simulink model "Q4_Simulink"  (R2019b)
settings: Solver=VariableStepAuto  StartTime=0.0  StopTime=simTime  RelTol=1e-3
values from neighbouring files (symbols this model uses):
  atan_scale = 100    [Q6.mat]    (also in Q8.mat)
  b_1 = 0.0029    [Q6.mat]    (also in Q8.mat)
  b_2 = 0.0002    [Q6.mat]    (also in Q8.mat)
  b_3 = 0.00015    [Q6.mat]    (also in Q8.mat)
  C = [1 0 0 0 0 0 0 1 0 0 0 0 ... (18 elements, 3x6)]    [Q6.mat]    (also in Q8.mat)
  f_m = 0.00325471482319    [Q6.mat]
  f_m_time = 5    [Q6.mat]
  J_1 = 0.0025    [Q6.mat]    (also in Q8.mat)
  J_2 = 0.0018    [Q6.mat]    (also in Q8.mat)
  J_3 = 0.0018    [Q6.mat]    (also in Q8.mat)
  k_1 = 2.7    [Q6.mat]    (also in Q8.mat)
  k_2 = 2.6    [Q6.mat]    (also in Q8.mat)
  switch_fault = 1    [Q6.mat]
  T_Cm = 0.0969711017207    [Q6.mat]    (also in Q8.mat)
  T_Cp = 0.0714454263135    [Q6.mat]    (also in Q8.mat)
  T_s = 0.004    [Q6.mat]
  w_th = 0.75    [Q6.mat]    (also in Q8.mat)
  wn = 1    [Q6.mat]
  x_0 = [0 0 0 0 0 0]    [Q6.mat]
  zeta = 0.96    [Q6.mat]
undefined symbols (not defined in the file or in its folder): den_tf_11, den_tf_21, num_tf_11, num_tf_21, sigma_meas
settings Model: Creator=mfust  LastModifiedBy=mfust
settings DataIOCC: ReturnWorkspaceOutputs=off
settings DebuggingCC: ArithmeticOperatorsInVariantConditions=warning
settings SFSimCC: SimUseLocalCustomCode=off  CustomCodeUndefinedFunction=UseInterfaceOnly
settings RTWCC: RTWUseLocalCustomCode=off

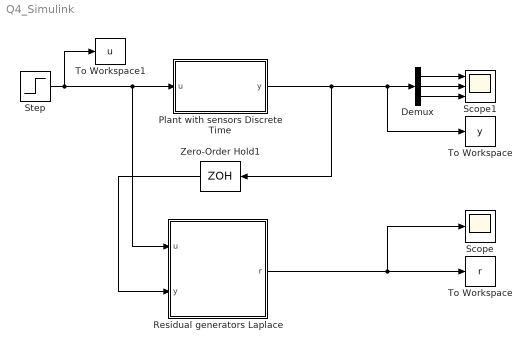
== system Q4_Simulink ==
  Demux : Demux  Outputs=3
  Plant with sensors Discrete Time : Subsystem
  Residual generators Laplace : Subsystem
  Scope : Scope
  Scope1 : Scope  NumInputPorts=3
  Step : Step  Time=2  SampleTime=0
  To Workspace : ToWorkspace  VariableName=y  SaveFormat=Structure With Time  SampleTime=-1
  "To Workspace " : ToWorkspace  VariableName=r  SaveFormat=Structure With Time  SampleTime=-1
  To Workspace1 : ToWorkspace  VariableName=u  SaveFormat=Structure With Time  SampleTime=-1
  Zero-Order Hold1 : ZeroOrderHold  SampleTime=T_s
  wires:
  Residual generators Laplace/1(r) -> Scope/1, "To Workspace "/1
  Step/1 -> Residual generators Laplace/1(u), Plant with sensors Discrete Time/1(u), To Workspace1/1
  Demux/1 -> Scope1/1
  Demux/2 -> Scope1/2
  Demux/3 -> Scope1/3
  Plant with sensors Discrete Time/1(y) -> Zero-Order Hold1/1, To Workspace/1, Demux/1
  Zero-Order Hold1/1 -> Residual generators Laplace/2(y)

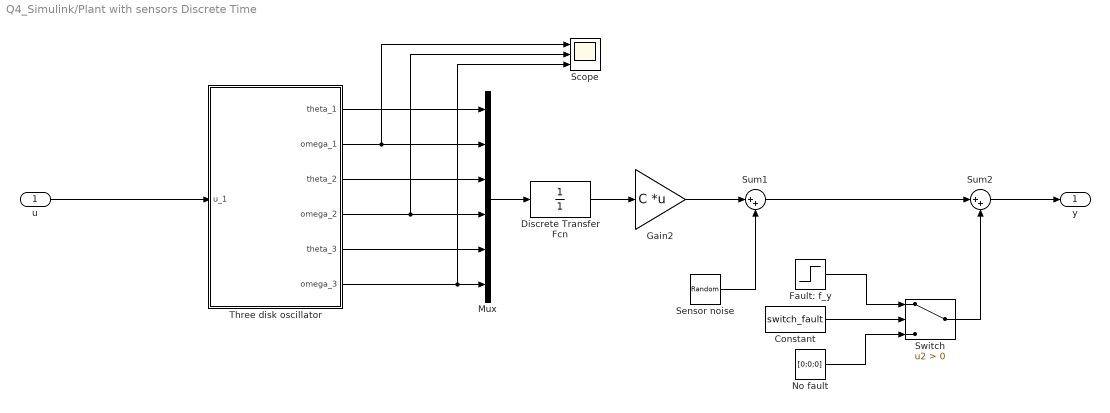
== system Q4_Simulink/Plant with sensors Discrete Time ==
  u : Inport
  Constant : Constant  Value=switch_fault
  Discrete Transfer Fcn : DiscreteTransferFcn  Denominator=[1]  SampleTime=T_s
  Fault: f_y : Step  Time=f_m_time  Before=[0;0;0]  After=f_m  SampleTime=0
  Gain2 : Gain  Gain=C  Multiplication=Matrix(K*u) (u vector)
  Mux : Mux  Inputs=6
  No fault : Constant  Value=[0;0;0]
  Scope : Scope  NumInputPorts=3
  Sensor noise : RandomNumber  Mean=zeros(3,1)  Variance=sigma_meas  SampleTime=T_s
  Sum1 : Sum  Inputs=|++
  Sum2 : Sum  Inputs=|++
  Switch : Switch  Criteria=u2 > Threshold
  Three disk oscillator : Subsystem
  y : Outport  VectorParamsAs1DForOutWhenUnconnected=off
  wires:
  u/1 -> Three disk oscillator/1(u_1)
  Three disk oscillator/2(omega_1) -> Scope/1, Mux/2
  Three disk oscillator/1(theta_1) -> Mux/1
  Mux/1 -> Discrete Transfer Fcn/1
  Three disk oscillator/4(omega_2) -> Scope/2, Mux/4
  Three disk oscillator/3(theta_2) -> Mux/3
  Discrete Transfer Fcn/1 -> Gain2/1
  Sum2/1 -> y/1
  Three disk oscillator/6(omega_3) -> Scope/3, Mux/6
  Three disk oscillator/5(theta_3) -> Mux/5
  Sum1/1 -> Sum2/1
  Gain2/1 -> Sum1/1
  Sensor noise/1 -> Sum1/2
  Switch/1 -> Sum2/2
  Constant/1 -> Switch/2
  Fault: f_y/1 -> Switch/1
  No fault/1 -> Switch/3

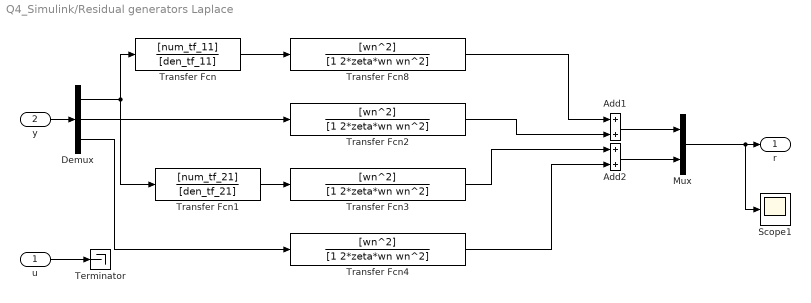
== system Q4_Simulink/Residual generators Laplace ==
  u : Inport
  y : Inport  Port=2
  Add1 : Sum
  Add2 : Sum
  Demux : Demux  Outputs=3
  Mux : Mux  Inputs=2
  Scope1 : Scope
  Terminator : Terminator
  Transfer Fcn : TransferFcn  Numerator=[num_tf_11]  Denominator=[den_tf_11]
  Transfer Fcn1 : TransferFcn  Numerator=[num_tf_21]  Denominator=[den_tf_21]
  Transfer Fcn{2..4,8} (4 alike) : TransferFcn  Numerator=[wn^2]  Denominator=[1 2*zeta*wn wn^2]
  r : Outport  VectorParamsAs1DForOutWhenUnconnected=off
  wires:
  Mux/1 -> Scope1/1, r/1
  y/1 -> Demux/1
  Demux/1 -> Transfer Fcn/1, Transfer Fcn1/1
  u/1 -> Terminator/1
  Add1/1 -> Mux/1
  Add2/1 -> Mux/2
  Transfer Fcn/1 -> Transfer Fcn8/1
  Transfer Fcn8/1 -> Add1/1
  Demux/2 -> Transfer Fcn2/1
  Transfer Fcn2/1 -> Add1/2
  Transfer Fcn1/1 -> Transfer Fcn3/1
  Transfer Fcn3/1 -> Add2/1
  Demux/3 -> Transfer Fcn4/1
  Transfer Fcn4/1 -> Add2/2

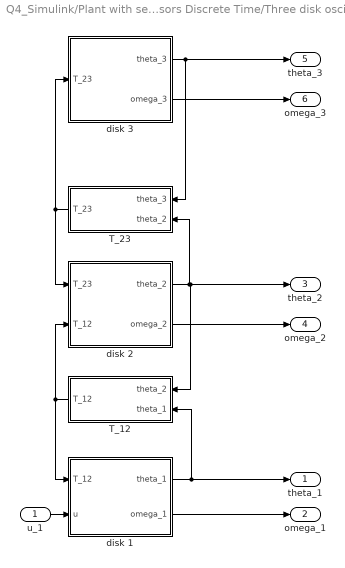
== system Q4_Simulink/Plant with sensors Discrete Time/Three disk oscillator ==
  u_1 : Inport
  T_12 : Subsystem
  T_23 : Subsystem
  disk 1 : Subsystem
  disk 2 : Subsystem
  disk 3 : Subsystem
  theta_1 : Outport  VectorParamsAs1DForOutWhenUnconnected=off
  omega_1 : Outport  Port=2  VectorParamsAs1DForOutWhenUnconnected=off
  theta_2 : Outport  Port=3  VectorParamsAs1DForOutWhenUnconnected=off
  omega_2 : Outport  Port=4  VectorParamsAs1DForOutWhenUnconnected=off
  theta_3 : Outport  Port=5  VectorParamsAs1DForOutWhenUnconnected=off
  omega_3 : Outport  Port=6  VectorParamsAs1DForOutWhenUnconnected=off
  wires:
  T_23/1(T_23) -> disk 2/1(T_23), disk 3/1(T_23)
  disk 1/1(theta_1) -> T_12/2(theta_1), theta_1/1
  disk 2/1(theta_2) -> T_23/2(theta_2), theta_2/1, T_12/1(theta_2)
  T_12/1(T_12) -> disk 1/1(T_12), disk 2/2(T_12)
  disk 3/2(omega_3) -> omega_3/1
  disk 1/2(omega_1) -> omega_1/1
  disk 2/2(omega_2) -> omega_2/1
  u_1/1 -> disk 1/2(u)
  disk 3/1(theta_3) -> theta_3/1, T_23/1(theta_3)

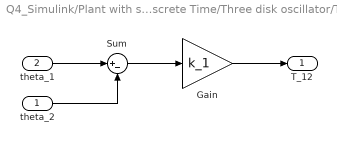
== system Q4_Simulink/Plant with sensors Discrete Time/Three disk oscillator/T_12 ==
  theta_2 : Inport
  theta_1 : Inport  Port=2
  Gain : Gain  Gain=k_1
  Sum : Sum  Inputs=|+-
  T_12 : Outport  VectorParamsAs1DForOutWhenUnconnected=off
  wires:
  theta_2/1 -> Sum/2
  theta_1/1 -> Sum/1
  Sum/1 -> Gain/1
  Gain/1 -> T_12/1

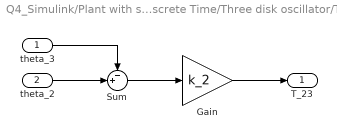
== system Q4_Simulink/Plant with sensors Discrete Time/Three disk oscillator/T_23 ==
  theta_3 : Inport
  theta_2 : Inport  Port=2
  Gain : Gain  Gain=k_2
  Sum : Sum  Inputs=-+|
  T_23 : Outport  VectorParamsAs1DForOutWhenUnconnected=off
  wires:
  Gain/1 -> T_23/1
  Sum/1 -> Gain/1
  theta_3/1 -> Sum/1
  theta_2/1 -> Sum/2

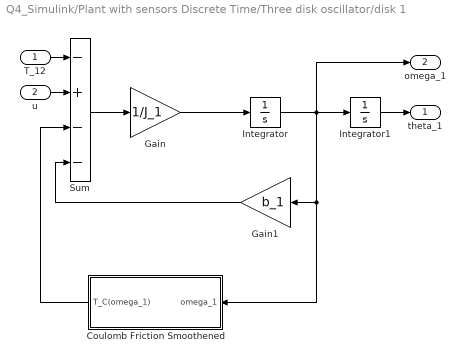
== system Q4_Simulink/Plant with sensors Discrete Time/Three disk oscillator/disk 1 ==
  T_12 : Inport
  u : Inport  Port=2
  Coulomb Friction Smoothened : Subsystem
  Gain : Gain  Gain=1/J_1
  Gain1 : Gain  Gain=b_1
  Integrator : Integrator  InitialCondition=x_0(2)
  Integrator1 : Integrator  InitialCondition=x_0(1)
  Sum : Sum  Inputs=-+--
  theta_1 : Outport  VectorParamsAs1DForOutWhenUnconnected=off
  omega_1 : Outport  Port=2  VectorParamsAs1DForOutWhenUnconnected=off
  wires:
  Sum/1 -> Gain/1
  Integrator/1 -> Integrator1/1, omega_1/1, Coulomb Friction Smoothened/1(omega_1), Gain1/1
  Gain1/1 -> Sum/4
  Integrator1/1 -> theta_1/1
  T_12/1 -> Sum/1
  u/1 -> Sum/2
  Gain/1 -> Integrator/1
  Coulomb Friction Smoothened/1(T_C(omega_1)) -> Sum/3

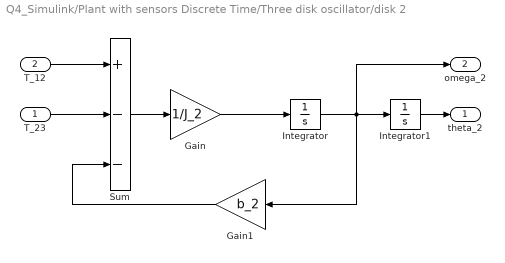
== system Q4_Simulink/Plant with sensors Discrete Time/Three disk oscillator/disk 2 ==
  T_23 : Inport
  T_12 : Inport  Port=2
  Gain : Gain  Gain=1/J_2
  Gain1 : Gain  Gain=b_2
  Integrator : Integrator  InitialCondition=x_0(4)
  Integrator1 : Integrator  InitialCondition=x_0(3)
  Sum : Sum  Inputs=+--
  theta_2 : Outport  VectorParamsAs1DForOutWhenUnconnected=off
  omega_2 : Outport  Port=2  VectorParamsAs1DForOutWhenUnconnected=off
  wires:
  T_23/1 -> Sum/2
  T_12/1 -> Sum/1
  Integrator1/1 -> theta_2/1
  Gain1/1 -> Sum/3
  Gain/1 -> Integrator/1
  Integrator/1 -> Integrator1/1, Gain1/1, omega_2/1
  Sum/1 -> Gain/1

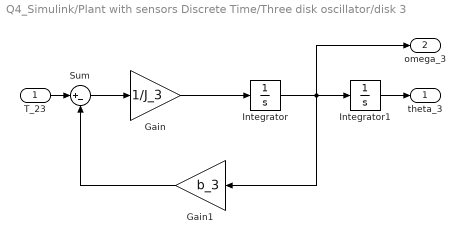
== system Q4_Simulink/Plant with sensors Discrete Time/Three disk oscillator/disk 3 ==
  T_23 : Inport
  Gain : Gain  Gain=1/J_3
  Gain1 : Gain  Gain=b_3
  Integrator : Integrator  InitialCondition=x_0(6)
  Integrator1 : Integrator  InitialCondition=x_0(5)
  Sum : Sum  Inputs=|+-
  theta_3 : Outport  VectorParamsAs1DForOutWhenUnconnected=off
  omega_3 : Outport  Port=2  VectorParamsAs1DForOutWhenUnconnected=off
  wires:
  Sum/1 -> Gain/1
  Integrator/1 -> Integrator1/1, omega_3/1, Gain1/1
  Gain/1 -> Integrator/1
  Gain1/1 -> Sum/2
  Integrator1/1 -> theta_3/1
  T_23/1 -> Sum/1

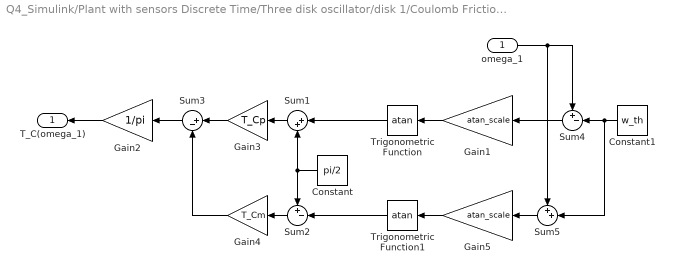
== system Q4_Simulink/Plant with sensors Discrete Time/Three disk oscillator/disk 1/Coulomb Friction Smoothened ==
  omega_1 : Inport
  Constant : Constant  Value=pi/2
  Constant1 : Constant  Value=w_th
  Gain1 : Gain  Gain=atan_scale
  Gain2 : Gain  Gain=1/pi
  Gain3 : Gain  Gain=T_Cp
  Gain4 : Gain  Gain=T_Cm
  Gain5 : Gain  Gain=atan_scale
  Sum1 : Sum  Inputs=|++
  Sum2 : Sum  Inputs=+-|
  Sum3 : Sum  Inputs=|+-
  Sum4 : Sum  Inputs=+-|
  Sum5 : Sum  Inputs=++|
  Trigonometric Function : Trigonometry  Operator=atan
  Trigonometric Function1 : Trigonometry  Operator=atan
  T_C(omega_1) : Outport  VectorParamsAs1DForOutWhenUnconnected=off
  wires:
  Gain1/1 -> Trigonometric Function/1
  Sum1/1 -> Gain3/1
  Constant/1 -> Sum2/1, Sum1/2
  Sum2/1 -> Gain4/1
  Sum3/1 -> Gain2/1
  Trigonometric Function/1 -> Sum1/1
  Gain4/1 -> Sum3/2
  Gain2/1 -> T_C(omega_1)/1
  omega_1/1 -> Sum5/1, Sum4/1
  Gain3/1 -> Sum3/1
  Sum4/1 -> Gain1/1
  Constant1/1 -> Sum5/2, Sum4/2
  Gain5/1 -> Trigonometric Function1/1
  Sum5/1 -> Gain5/1
  Trigonometric Function1/1 -> Sum2/2
